simulink model "Problem_8"  (R2020a)
settings: Solver=VariableStepAuto  StartTime=0.0  StopTime=5  RelTol=1e-3
settings Model: EnablePacing=on  PacingRate=0.450000  Creator=Ganesh  LastModifiedBy=Avengers

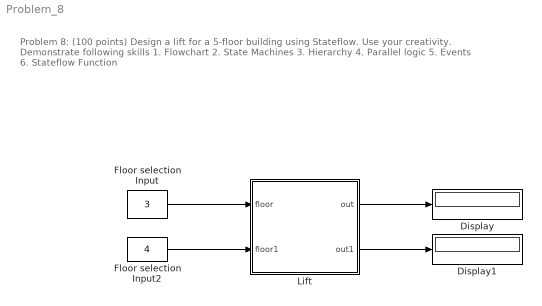
== system Problem_8 ==
  note: Problem 8: (100 points) Design a lift for a 5-floor building using Stateflow. Use your creativity.
      | Demonstrate following skills
      | 1. Flowchart
      | 2. State Machines
      | 3. Hierarchy
      | 4. Parallel logic
      | 5. Events
      | 6. Stateflow Function
  Display : Display
  Display1 : Display
  Floor selection Input : Constant  Value=3
  Floor selection Input2 : Constant  Value=4
  Lift : Stateflow chart  TreatAsAtomicUnit=on
  wires:
  Floor selection Input2/1 -> Lift/2(floor1)
  Lift/1(out) -> Display/1
  Lift/2(out1) -> Display1/1
  Floor selection Input/1 -> Lift/1(floor)

== stateflow chart Problem_8/Lift ==
  state Start
    (history)
    state Lift_For_five_floor
      (history)
      state Floor1
        entry:
        present=1;
        out=1;
      state Floor2
        entry:
        out=2;
        present=out;
      state Floor3
        entry:
        out=3;
        present=out;
      state Floor4
        entry:
        out=4;
        present=out;
      state Floor5
        entry:
        out=5;
        present=out
      Start.Lift_For_five_floor.Floor1 -> Start.Lift_For_five_floor.Floor1 [order 2] : [present==floor]
      (default) -> Start.Lift_For_five_floor.Floor1
      Start.Lift_For_five_floor.Floor3 -> Start.Lift_For_five_floor.Floor4 [order 1] : [present<floor]
      Start.Lift_For_five_floor.Floor2 -> Start.Lift_For_five_floor.Floor3 [order 1] : [present<floor]
      Start.Lift_For_five_floor.Floor4 -> Start.Lift_For_five_floor.Floor5 [order 1] : [present<floor]
      Start.Lift_For_five_floor.Floor1 -> Start.Lift_For_five_floor.Floor2 [order 1] : [present<floor]
      Start.Lift_For_five_floor.Floor5 -> Start.Lift_For_five_floor.Floor5 [order 2] : [floor==present]
      Start.Lift_For_five_floor.Floor5 -> Start.Lift_For_five_floor.Floor4 [order 1] : [present>floor]
      Start.Lift_For_five_floor.Floor4 -> Start.Lift_For_five_floor.Floor3 [order 2] : [present>floor]
      Start.Lift_For_five_floor.Floor2 -> Start.Lift_For_five_floor.Floor1 [order 2] : [present>floor]
      Start.Lift_For_five_floor.Floor3 -> Start.Lift_For_five_floor.Floor2 [order 2] : [present>floor]
    state Second_input
      (history)
      state Floor1
        entry:
        present=1;
        out1=1;
      state Floor2
        entry:
        out1=2;
        present=out1;
      state Floor3
        entry:
        out1=3;
        present=out1;
      state Floor4
        entry:
        out1=4;
        present=out1;
      state Floor5
        entry:
        out1=5;
        present=out1;
      Start.Second_input.Floor1 -> Start.Second_input.Floor1 [order 2] : [present==floor1]
      (default) -> Start.Second_input.Floor1
      Start.Second_input.Floor3 -> Start.Second_input.Floor4 [order 1] : [present<floor1]
      Start.Second_input.Floor2 -> Start.Second_input.Floor3 [order 1] : [present<floor1]
      Start.Second_input.Floor4 -> Start.Second_input.Floor5 [order 1] : [present<floor1]
      Start.Second_input.Floor1 -> Start.Second_input.Floor2 [order 1] : [present<floor1]
      Start.Second_input.Floor5 -> Start.Second_input.Floor5 [order 2] : [floor==present]
      Start.Second_input.Floor5 -> Start.Second_input.Floor4 [order 1] : [present>floor1]
      Start.Second_input.Floor4 -> Start.Second_input.Floor3 [order 2] : [present>floor1]
      Start.Second_input.Floor2 -> Start.Second_input.Floor1 [order 2] : [present>floor1]
      Start.Second_input.Floor3 -> Start.Second_input.Floor2 [order 2] : [present>floor1]
    (default) -> Lift_For_five_floor
    Lift_For_five_floor -> Second_input : [present==floor]
  (default) -> Start
  data: floor input; present local; out output; floor1 input; out1 output
